simulink model "spoco6_250"  (R2013a)
settings: Solver=VariableStepDiscrete  SolverMode=SingleTasking  StartTime=0.0  StopTime=10.0  RelTol=1e-3
undefined symbols (not defined in the file or in its folder): casper_library_multipliers, cmult_4bit_em
libraries: xbsIndex_r4 x1937, xps_library x51, casper_library_misc x45, casper_library_sources x6
(part 8 of 23)

== system spoco6_250/xengine6/af ==
  a+bi : Inport
  c+di : Inport  Port=2
  new_acc : Inport  Port=3
  Counter : xbsIndex_r4/Counter  cnt_type=Free Running  cnt_to=Inf  operation=Up  start_count=0  cnt_by_val=1  arith_type=Unsigned  n_bits=nchan  bin_pt=0  load_pin=off  rst=on  en=on  explicit_period=on  period=1  use_behavioral_HDL=off  implementation=Fabric  dbl_ovrd=off  block_type=counter
  Delay : xbsIndex_r4/Delay  rst=off  infoeditControl=Selection of Reset will increase slice count due to use of real FFs and instead of SRLs  en=off  latency=mult_latency + add_latency  reg_retiming=off  dbl_ovrd=off  block_type=delay
  c_to_ri1 : casper_library_misc/c_to_ri  n_bits=n_bits  bin_pt=n_bits-1
      settings: AttributesFormatString=4_3 r/i
  c_to_ri2 : casper_library_misc/c_to_ri  n_bits=n_bits  bin_pt=n_bits-1
      settings: AttributesFormatString=4_3 r/i
  cmult_4bit_em* : Subsystem  AncestorBlock=casper_library_multipliers/cmult_4bit_em*  mask(cmult_4bit_em*){mult_latency=mult_latency, add_latency=add_latency}
      mask prompts: mult_latency "Mult Latency"; add_latency "Add Latency"
      mask help: Perform a conjugating complex multiplication (a+bi)(c-di)=(ac+bd)+(bc-ad)i. Implements the logic in dedicated multipliers.
      mask Help: eval('xlWeb(''http://casper.berkeley.edu/wiki/Cmult_4bit_em_'')')
  imag : xps_library/Shared BRAM  Tag=xps:bram  arith_type="Signed  (2's comp)"  addr_width=max(nchan,10)  data_width=32  reg_prim_output=off  reg_core_output=off  optimization=Minimum_Area  data_bin_pt=min(2*(n_bits-1), 30)  init_vals=0  sample_rate=1
  real : xps_library/Shared BRAM  Tag=xps:bram  arith_type="Signed  (2's comp)"  addr_width=max(nchan,10)  data_width=32  reg_prim_output=off  reg_core_output=off  optimization=Minimum_Area  data_bin_pt=min(2*(n_bits-1), 30)  init_vals=0  sample_rate=1
  simple_bram_vacc : Subsystem  AncestorBlock=casper_library_accumulators/simple_bram_vacc  mask(simple_bram_vacc){vec_len=2^nchan, arith_type=Signed, n_bits=32, bin_pt=30}
      mask prompts: vec_len "Vector length:"; arith_type "Output type:"; n_bits "Bit width (output):"; bin_pt "Binary point (output):"
      mask help: This simple vector accumulator is based on a shift register. It outputs its previous accumulated vector after a new_acc pulse is received.
      mask init:
      | simple_bram_vacc_init(gcb, ...
      |     'vec_len', vec_len, ...
      |     'arith_type', arith_type, ...
      |     'n_bits', n_bits, ...
      |     'bin_pt', bin_pt);
      mask TypeOptions arith_type: Signed | Unsigned
  simple_bram_vacc1 : Subsystem  AncestorBlock=casper_library_accumulators/simple_bram_vacc  mask(simple_bram_vacc){vec_len=2^nchan, arith_type=Signed, n_bits=32, bin_pt=30}
      mask prompts: vec_len "Vector length:"; arith_type "Output type:"; n_bits "Bit width (output):"; bin_pt "Binary point (output):"
      mask help: This simple vector accumulator is based on a shift register. It outputs its previous accumulated vector after a new_acc pulse is received.
      mask init:
      | simple_bram_vacc_init(gcb, ...
      |     'vec_len', vec_len, ...
      |     'arith_type', arith_type, ...
      |     'n_bits', n_bits, ...
      |     'bin_pt', bin_pt);
      mask TypeOptions arith_type: Signed | Unsigned
  wires:
  simple_bram_vacc1/2(valid) -> imag/3
  simple_bram_vacc1/1(dout) -> imag/2
  Delay/1 -> simple_bram_vacc1/1(new_acc), simple_bram_vacc/1(new_acc), Counter/1
  simple_bram_vacc/1(dout) -> real/2
  Counter/1 -> imag/1, real/1
  simple_bram_vacc/2(valid) -> Counter/2, real/3
  new_acc/1 -> Delay/1
  c+di/1 -> c_to_ri2/1
  a+bi/1 -> c_to_ri1/1
  c_to_ri1/1 -> cmult_4bit_em*/1(a)
  c_to_ri1/2 -> cmult_4bit_em*/2(b)
  c_to_ri2/2 -> cmult_4bit_em*/4(d)
  c_to_ri2/1 -> cmult_4bit_em*/3(c)
  cmult_4bit_em*/1(real) -> simple_bram_vacc/2(din)
  cmult_4bit_em*/2(imag) -> simple_bram_vacc1/2(din)

== system spoco6_250/xengine6/bb ==
  a+bi : Inport
  c+di : Inport  Port=2
  new_acc : Inport  Port=3
  Counter : xbsIndex_r4/Counter  cnt_type=Free Running  cnt_to=Inf  operation=Up  start_count=0  cnt_by_val=1  arith_type=Unsigned  n_bits=nchan  bin_pt=0  load_pin=off  rst=on  en=on  explicit_period=on  period=1  use_behavioral_HDL=off  implementation=Fabric  dbl_ovrd=off  block_type=counter
  Delay : xbsIndex_r4/Delay  rst=off  infoeditControl=Selection of Reset will increase slice count due to use of real FFs and instead of SRLs  en=off  latency=mult_latency + add_latency  reg_retiming=off  dbl_ovrd=off  block_type=delay
  c_to_ri1 : casper_library_misc/c_to_ri  n_bits=n_bits  bin_pt=n_bits-1
      settings: AttributesFormatString=4_3 r/i
  c_to_ri2 : casper_library_misc/c_to_ri  n_bits=n_bits  bin_pt=n_bits-1
      settings: AttributesFormatString=4_3 r/i
  cmult_4bit_em* : Subsystem  AncestorBlock=casper_library_multipliers/cmult_4bit_em*  mask(cmult_4bit_em*){mult_latency=mult_latency, add_latency=add_latency}
      mask prompts: mult_latency "Mult Latency"; add_latency "Add Latency"
      mask help: Perform a conjugating complex multiplication (a+bi)(c-di)=(ac+bd)+(bc-ad)i. Implements the logic in dedicated multipliers.
      mask Help: eval('xlWeb(''http://casper.berkeley.edu/wiki/Cmult_4bit_em_'')')
  real : xps_library/Shared BRAM  Tag=xps:bram  arith_type="Signed  (2's comp)"  addr_width=max(nchan,10)  data_width=32  reg_prim_output=off  reg_core_output=off  optimization=Minimum_Area  data_bin_pt=min(2*(n_bits-1), 30)  init_vals=0  sample_rate=1
  simple_bram_vacc : Subsystem  AncestorBlock=casper_library_accumulators/simple_bram_vacc  mask(simple_bram_vacc){vec_len=2^nchan, arith_type=Signed, n_bits=32, bin_pt=30}
      mask prompts: vec_len "Vector length:"; arith_type "Output type:"; n_bits "Bit width (output):"; bin_pt "Binary point (output):"
      mask help: This simple vector accumulator is based on a shift register. It outputs its previous accumulated vector after a new_acc pulse is received.
      mask init:
      | simple_bram_vacc_init(gcb, ...
      |     'vec_len', vec_len, ...
      |     'arith_type', arith_type, ...
      |     'n_bits', n_bits, ...
      |     'bin_pt', bin_pt);
      mask TypeOptions arith_type: Signed | Unsigned
  wires:
  c_to_ri2/1 -> cmult_4bit_em*/3(c)
  c_to_ri2/2 -> cmult_4bit_em*/4(d)
  c_to_ri1/2 -> cmult_4bit_em*/2(b)
  c_to_ri1/1 -> cmult_4bit_em*/1(a)
  Delay/1 -> simple_bram_vacc/1(new_acc), Counter/1
  simple_bram_vacc/1(dout) -> real/2
  Counter/1 -> real/1
  simple_bram_vacc/2(valid) -> real/3, Counter/2
  a+bi/1 -> c_to_ri1/1
  c+di/1 -> c_to_ri2/1
  new_acc/1 -> Delay/1
  cmult_4bit_em*/1(real) -> simple_bram_vacc/2(din)

== system spoco6_250/xengine6/bc ==
  a+bi : Inport
  c+di : Inport  Port=2
  new_acc : Inport  Port=3
  Counter : xbsIndex_r4/Counter  cnt_type=Free Running  cnt_to=Inf  operation=Up  start_count=0  cnt_by_val=1  arith_type=Unsigned  n_bits=nchan  bin_pt=0  load_pin=off  rst=on  en=on  explicit_period=on  period=1  use_behavioral_HDL=off  implementation=Fabric  dbl_ovrd=off  block_type=counter
  Delay : xbsIndex_r4/Delay  rst=off  infoeditControl=Selection of Reset will increase slice count due to use of real FFs and instead of SRLs  en=off  latency=mult_latency + add_latency  reg_retiming=off  dbl_ovrd=off  block_type=delay
  c_to_ri1 : casper_library_misc/c_to_ri  n_bits=n_bits  bin_pt=n_bits-1
      settings: AttributesFormatString=4_3 r/i
  c_to_ri2 : casper_library_misc/c_to_ri  n_bits=n_bits  bin_pt=n_bits-1
      settings: AttributesFormatString=4_3 r/i
  cmult_4bit_em* : Subsystem  AncestorBlock=casper_library_multipliers/cmult_4bit_em*  mask(cmult_4bit_em*){mult_latency=mult_latency, add_latency=add_latency}
      mask prompts: mult_latency "Mult Latency"; add_latency "Add Latency"
      mask help: Perform a conjugating complex multiplication (a+bi)(c-di)=(ac+bd)+(bc-ad)i. Implements the logic in dedicated multipliers.
      mask Help: eval('xlWeb(''http://casper.berkeley.edu/wiki/Cmult_4bit_em_'')')
  imag : xps_library/Shared BRAM  Tag=xps:bram  arith_type="Signed  (2's comp)"  addr_width=max(nchan,10)  data_width=32  reg_prim_output=off  reg_core_output=off  optimization=Minimum_Area  data_bin_pt=min(2*(n_bits-1), 30)  init_vals=0  sample_rate=1
  real : xps_library/Shared BRAM  Tag=xps:bram  arith_type="Signed  (2's comp)"  addr_width=max(nchan,10)  data_width=32  reg_prim_output=off  reg_core_output=off  optimization=Minimum_Area  data_bin_pt=min(2*(n_bits-1), 30)  init_vals=0  sample_rate=1
  simple_bram_vacc : Subsystem  AncestorBlock=casper_library_accumulators/simple_bram_vacc  mask(simple_bram_vacc){vec_len=2^nchan, arith_type=Signed, n_bits=32, bin_pt=30}
      mask prompts: vec_len "Vector length:"; arith_type "Output type:"; n_bits "Bit width (output):"; bin_pt "Binary point (output):"
      mask help: This simple vector accumulator is based on a shift register. It outputs its previous accumulated vector after a new_acc pulse is received.
      mask init:
      | simple_bram_vacc_init(gcb, ...
      |     'vec_len', vec_len, ...
      |     'arith_type', arith_type, ...
      |     'n_bits', n_bits, ...
      |     'bin_pt', bin_pt);
      mask TypeOptions arith_type: Signed | Unsigned
  simple_bram_vacc1 : Subsystem  AncestorBlock=casper_library_accumulators/simple_bram_vacc  mask(simple_bram_vacc){vec_len=2^nchan, arith_type=Signed, n_bits=32, bin_pt=30}
      mask prompts: vec_len "Vector length:"; arith_type "Output type:"; n_bits "Bit width (output):"; bin_pt "Binary point (output):"
      mask help: This simple vector accumulator is based on a shift register. It outputs its previous accumulated vector after a new_acc pulse is received.
      mask init:
      | simple_bram_vacc_init(gcb, ...
      |     'vec_len', vec_len, ...
      |     'arith_type', arith_type, ...
      |     'n_bits', n_bits, ...
      |     'bin_pt', bin_pt);
      mask TypeOptions arith_type: Signed | Unsigned
  wires:
  simple_bram_vacc1/2(valid) -> imag/3
  simple_bram_vacc1/1(dout) -> imag/2
  Delay/1 -> simple_bram_vacc1/1(new_acc), simple_bram_vacc/1(new_acc), Counter/1
  simple_bram_vacc/1(dout) -> real/2
  Counter/1 -> imag/1, real/1
  simple_bram_vacc/2(valid) -> Counter/2, real/3
  new_acc/1 -> Delay/1
  c+di/1 -> c_to_ri2/1
  a+bi/1 -> c_to_ri1/1
  c_to_ri1/1 -> cmult_4bit_em*/1(a)
  c_to_ri1/2 -> cmult_4bit_em*/2(b)
  c_to_ri2/2 -> cmult_4bit_em*/4(d)
  c_to_ri2/1 -> cmult_4bit_em*/3(c)
  cmult_4bit_em*/1(real) -> simple_bram_vacc/2(din)
  cmult_4bit_em*/2(imag) -> simple_bram_vacc1/2(din)

== system spoco6_250/xengine6/bd ==
  a+bi : Inport
  c+di : Inport  Port=2
  new_acc : Inport  Port=3
  Counter : xbsIndex_r4/Counter  cnt_type=Free Running  cnt_to=Inf  operation=Up  start_count=0  cnt_by_val=1  arith_type=Unsigned  n_bits=nchan  bin_pt=0  load_pin=off  rst=on  en=on  explicit_period=on  period=1  use_behavioral_HDL=off  implementation=Fabric  dbl_ovrd=off  block_type=counter
  Delay : xbsIndex_r4/Delay  rst=off  infoeditControl=Selection of Reset will increase slice count due to use of real FFs and instead of SRLs  en=off  latency=mult_latency + add_latency  reg_retiming=off  dbl_ovrd=off  block_type=delay
  c_to_ri1 : casper_library_misc/c_to_ri  n_bits=n_bits  bin_pt=n_bits-1
      settings: AttributesFormatString=4_3 r/i
  c_to_ri2 : casper_library_misc/c_to_ri  n_bits=n_bits  bin_pt=n_bits-1
      settings: AttributesFormatString=4_3 r/i
  cmult_4bit_em* : Subsystem  AncestorBlock=casper_library_multipliers/cmult_4bit_em*  mask(cmult_4bit_em*){mult_latency=mult_latency, add_latency=add_latency}
      mask prompts: mult_latency "Mult Latency"; add_latency "Add Latency"
      mask help: Perform a conjugating complex multiplication (a+bi)(c-di)=(ac+bd)+(bc-ad)i. Implements the logic in dedicated multipliers.
      mask Help: eval('xlWeb(''http://casper.berkeley.edu/wiki/Cmult_4bit_em_'')')
  imag : xps_library/Shared BRAM  Tag=xps:bram  arith_type="Signed  (2's comp)"  addr_width=max(nchan,10)  data_width=32  reg_prim_output=off  reg_core_output=off  optimization=Minimum_Area  data_bin_pt=min(2*(n_bits-1), 30)  init_vals=0  sample_rate=1
  real : xps_library/Shared BRAM  Tag=xps:bram  arith_type="Signed  (2's comp)"  addr_width=max(nchan,10)  data_width=32  reg_prim_output=off  reg_core_output=off  optimization=Minimum_Area  data_bin_pt=min(2*(n_bits-1), 30)  init_vals=0  sample_rate=1
  simple_bram_vacc : Subsystem  AncestorBlock=casper_library_accumulators/simple_bram_vacc  mask(simple_bram_vacc){vec_len=2^nchan, arith_type=Signed, n_bits=32, bin_pt=30}
      mask prompts: vec_len "Vector length:"; arith_type "Output type:"; n_bits "Bit width (output):"; bin_pt "Binary point (output):"
      mask help: This simple vector accumulator is based on a shift register. It outputs its previous accumulated vector after a new_acc pulse is received.
      mask init:
      | simple_bram_vacc_init(gcb, ...
      |     'vec_len', vec_len, ...
      |     'arith_type', arith_type, ...
      |     'n_bits', n_bits, ...
      |     'bin_pt', bin_pt);
      mask TypeOptions arith_type: Signed | Unsigned
  simple_bram_vacc1 : Subsystem  AncestorBlock=casper_library_accumulators/simple_bram_vacc  mask(simple_bram_vacc){vec_len=2^nchan, arith_type=Signed, n_bits=32, bin_pt=30}
      mask prompts: vec_len "Vector length:"; arith_type "Output type:"; n_bits "Bit width (output):"; bin_pt "Binary point (output):"
      mask help: This simple vector accumulator is based on a shift register. It outputs its previous accumulated vector after a new_acc pulse is received.
      mask init:
      | simple_bram_vacc_init(gcb, ...
      |     'vec_len', vec_len, ...
      |     'arith_type', arith_type, ...
      |     'n_bits', n_bits, ...
      |     'bin_pt', bin_pt);
      mask TypeOptions arith_type: Signed | Unsigned
  wires:
  cmult_4bit_em*/2(imag) -> simple_bram_vacc1/2(din)
  cmult_4bit_em*/1(real) -> simple_bram_vacc/2(din)
  c_to_ri2/1 -> cmult_4bit_em*/3(c)
  c_to_ri2/2 -> cmult_4bit_em*/4(d)
  c_to_ri1/2 -> cmult_4bit_em*/2(b)
  c_to_ri1/1 -> cmult_4bit_em*/1(a)
  a+bi/1 -> c_to_ri1/1
  c+di/1 -> c_to_ri2/1
  new_acc/1 -> Delay/1
  simple_bram_vacc/2(valid) -> real/3, Counter/2
  Counter/1 -> real/1, imag/1
  simple_bram_vacc/1(dout) -> real/2
  Delay/1 -> Counter/1, simple_bram_vacc/1(new_acc), simple_bram_vacc1/1(new_acc)
  simple_bram_vacc1/1(dout) -> imag/2
  simple_bram_vacc1/2(valid) -> imag/3

== system spoco6_250/xengine6/be ==
  a+bi : Inport
  c+di : Inport  Port=2
  new_acc : Inport  Port=3
  Counter : xbsIndex_r4/Counter  cnt_type=Free Running  cnt_to=Inf  operation=Up  start_count=0  cnt_by_val=1  arith_type=Unsigned  n_bits=nchan  bin_pt=0  load_pin=off  rst=on  en=on  explicit_period=on  period=1  use_behavioral_HDL=off  implementation=Fabric  dbl_ovrd=off  block_type=counter
  Delay : xbsIndex_r4/Delay  rst=off  infoeditControl=Selection of Reset will increase slice count due to use of real FFs and instead of SRLs  en=off  latency=mult_latency + add_latency  reg_retiming=off  dbl_ovrd=off  block_type=delay
  c_to_ri1 : casper_library_misc/c_to_ri  n_bits=n_bits  bin_pt=n_bits-1
      settings: AttributesFormatString=4_3 r/i
  c_to_ri2 : casper_library_misc/c_to_ri  n_bits=n_bits  bin_pt=n_bits-1
      settings: AttributesFormatString=4_3 r/i
  cmult_4bit_em* : Subsystem  AncestorBlock=casper_library_multipliers/cmult_4bit_em*  mask(cmult_4bit_em*){mult_latency=mult_latency, add_latency=add_latency}
      mask prompts: mult_latency "Mult Latency"; add_latency "Add Latency"
      mask help: Perform a conjugating complex multiplication (a+bi)(c-di)=(ac+bd)+(bc-ad)i. Implements the logic in dedicated multipliers.
      mask Help: eval('xlWeb(''http://casper.berkeley.edu/wiki/Cmult_4bit_em_'')')
  imag : xps_library/Shared BRAM  Tag=xps:bram  arith_type="Signed  (2's comp)"  addr_width=max(nchan,10)  data_width=32  reg_prim_output=off  reg_core_output=off  optimization=Minimum_Area  data_bin_pt=min(2*(n_bits-1), 30)  init_vals=0  sample_rate=1
  real : xps_library/Shared BRAM  Tag=xps:bram  arith_type="Signed  (2's comp)"  addr_width=max(nchan,10)  data_width=32  reg_prim_output=off  reg_core_output=off  optimization=Minimum_Area  data_bin_pt=min(2*(n_bits-1), 30)  init_vals=0  sample_rate=1
  simple_bram_vacc : Subsystem  AncestorBlock=casper_library_accumulators/simple_bram_vacc  mask(simple_bram_vacc){vec_len=2^nchan, arith_type=Signed, n_bits=32, bin_pt=30}
      mask prompts: vec_len "Vector length:"; arith_type "Output type:"; n_bits "Bit width (output):"; bin_pt "Binary point (output):"
      mask help: This simple vector accumulator is based on a shift register. It outputs its previous accumulated vector after a new_acc pulse is received.
      mask init:
      | simple_bram_vacc_init(gcb, ...
      |     'vec_len', vec_len, ...
      |     'arith_type', arith_type, ...
      |     'n_bits', n_bits, ...
      |     'bin_pt', bin_pt);
      mask TypeOptions arith_type: Signed | Unsigned
  simple_bram_vacc1 : Subsystem  AncestorBlock=casper_library_accumulators/simple_bram_vacc  mask(simple_bram_vacc){vec_len=2^nchan, arith_type=Signed, n_bits=32, bin_pt=30}
      mask prompts: vec_len "Vector length:"; arith_type "Output type:"; n_bits "Bit width (output):"; bin_pt "Binary point (output):"
      mask help: This simple vector accumulator is based on a shift register. It outputs its previous accumulated vector after a new_acc pulse is received.
      mask init:
      | simple_bram_vacc_init(gcb, ...
      |     'vec_len', vec_len, ...
      |     'arith_type', arith_type, ...
      |     'n_bits', n_bits, ...
      |     'bin_pt', bin_pt);
      mask TypeOptions arith_type: Signed | Unsigned
  wires:
  simple_bram_vacc1/2(valid) -> imag/3
  simple_bram_vacc1/1(dout) -> imag/2
  Delay/1 -> simple_bram_vacc1/1(new_acc), simple_bram_vacc/1(new_acc), Counter/1
  simple_bram_vacc/1(dout) -> real/2
  Counter/1 -> imag/1, real/1
  simple_bram_vacc/2(valid) -> Counter/2, real/3
  new_acc/1 -> Delay/1
  c+di/1 -> c_to_ri2/1
  a+bi/1 -> c_to_ri1/1
  c_to_ri1/1 -> cmult_4bit_em*/1(a)
  c_to_ri1/2 -> cmult_4bit_em*/2(b)
  c_to_ri2/2 -> cmult_4bit_em*/4(d)
  c_to_ri2/1 -> cmult_4bit_em*/3(c)
  cmult_4bit_em*/1(real) -> simple_bram_vacc/2(din)
  cmult_4bit_em*/2(imag) -> simple_bram_vacc1/2(din)

== system spoco6_250/xengine6/bf ==
  a+bi : Inport
  c+di : Inport  Port=2
  new_acc : Inport  Port=3
  Counter : xbsIndex_r4/Counter  cnt_type=Free Running  cnt_to=Inf  operation=Up  start_count=0  cnt_by_val=1  arith_type=Unsigned  n_bits=nchan  bin_pt=0  load_pin=off  rst=on  en=on  explicit_period=on  period=1  use_behavioral_HDL=off  implementation=Fabric  dbl_ovrd=off  block_type=counter
  Delay : xbsIndex_r4/Delay  rst=off  infoeditControl=Selection of Reset will increase slice count due to use of real FFs and instead of SRLs  en=off  latency=mult_latency + add_latency  reg_retiming=off  dbl_ovrd=off  block_type=delay
  c_to_ri1 : casper_library_misc/c_to_ri  n_bits=n_bits  bin_pt=n_bits-1
      settings: AttributesFormatString=4_3 r/i
  c_to_ri2 : casper_library_misc/c_to_ri  n_bits=n_bits  bin_pt=n_bits-1
      settings: AttributesFormatString=4_3 r/i
  cmult_4bit_em* : Subsystem  AncestorBlock=casper_library_multipliers/cmult_4bit_em*  mask(cmult_4bit_em*){mult_latency=mult_latency, add_latency=add_latency}
      mask prompts: mult_latency "Mult Latency"; add_latency "Add Latency"
      mask help: Perform a conjugating complex multiplication (a+bi)(c-di)=(ac+bd)+(bc-ad)i. Implements the logic in dedicated multipliers.
      mask Help: eval('xlWeb(''http://casper.berkeley.edu/wiki/Cmult_4bit_em_'')')
  imag : xps_library/Shared BRAM  Tag=xps:bram  arith_type="Signed  (2's comp)"  addr_width=max(nchan,10)  data_width=32  reg_prim_output=off  reg_core_output=off  optimization=Minimum_Area  data_bin_pt=min(2*(n_bits-1), 30)  init_vals=0  sample_rate=1
  real : xps_library/Shared BRAM  Tag=xps:bram  arith_type="Signed  (2's comp)"  addr_width=max(nchan,10)  data_width=32  reg_prim_output=off  reg_core_output=off  optimization=Minimum_Area  data_bin_pt=min(2*(n_bits-1), 30)  init_vals=0  sample_rate=1
  simple_bram_vacc : Subsystem  AncestorBlock=casper_library_accumulators/simple_bram_vacc  mask(simple_bram_vacc){vec_len=2^nchan, arith_type=Signed, n_bits=32, bin_pt=30}
      mask prompts: vec_len "Vector length:"; arith_type "Output type:"; n_bits "Bit width (output):"; bin_pt "Binary point (output):"
      mask help: This simple vector accumulator is based on a shift register. It outputs its previous accumulated vector after a new_acc pulse is received.
      mask init:
      | simple_bram_vacc_init(gcb, ...
      |     'vec_len', vec_len, ...
      |     'arith_type', arith_type, ...
      |     'n_bits', n_bits, ...
      |     'bin_pt', bin_pt);
      mask TypeOptions arith_type: Signed | Unsigned
  simple_bram_vacc1 : Subsystem  AncestorBlock=casper_library_accumulators/simple_bram_vacc  mask(simple_bram_vacc){vec_len=2^nchan, arith_type=Signed, n_bits=32, bin_pt=30}
      mask prompts: vec_len "Vector length:"; arith_type "Output type:"; n_bits "Bit width (output):"; bin_pt "Binary point (output):"
      mask help: This simple vector accumulator is based on a shift register. It outputs its previous accumulated vector after a new_acc pulse is received.
      mask init:
      | simple_bram_vacc_init(gcb, ...
      |     'vec_len', vec_len, ...
      |     'arith_type', arith_type, ...
      |     'n_bits', n_bits, ...
      |     'bin_pt', bin_pt);
      mask TypeOptions arith_type: Signed | Unsigned
  wires:
  cmult_4bit_em*/2(imag) -> simple_bram_vacc1/2(din)
  cmult_4bit_em*/1(real) -> simple_bram_vacc/2(din)
  c_to_ri2/1 -> cmult_4bit_em*/3(c)
  c_to_ri2/2 -> cmult_4bit_em*/4(d)
  c_to_ri1/2 -> cmult_4bit_em*/2(b)
  c_to_ri1/1 -> cmult_4bit_em*/1(a)
  a+bi/1 -> c_to_ri1/1
  c+di/1 -> c_to_ri2/1
  new_acc/1 -> Delay/1
  simple_bram_vacc/2(valid) -> real/3, Counter/2
  Counter/1 -> real/1, imag/1
  simple_bram_vacc/1(dout) -> real/2
  Delay/1 -> Counter/1, simple_bram_vacc/1(new_acc), simple_bram_vacc1/1(new_acc)
  simple_bram_vacc1/1(dout) -> imag/2
  simple_bram_vacc1/2(valid) -> imag/3

== system spoco6_250/xengine6/bus_expand ==
  bus_in : Inport
  reinterpret{1..6} (6 alike) : xbsIndex_r4/Reinterpret  force_arith_type=on  arith_type=Unsigned  force_bin_pt=on  bin_pt=0  block_type=reinterpret
  slice1 : xbsIndex_r4/Slice  nbits=8  boolean_output=off  mode=Upper Bit Location + Width  bit1=-40  base1=MSB of Input  bit0=0  base0=LSB of Input  dbl_ovrd=off  block_type=slice
  slice2 : xbsIndex_r4/Slice  nbits=8  boolean_output=off  mode=Upper Bit Location + Width  bit1=-32  base1=MSB of Input  bit0=0  base0=LSB of Input  dbl_ovrd=off  block_type=slice
  slice3 : xbsIndex_r4/Slice  nbits=8  boolean_output=off  mode=Upper Bit Location + Width  bit1=-24  base1=MSB of Input  bit0=0  base0=LSB of Input  dbl_ovrd=off  block_type=slice
  slice4 : xbsIndex_r4/Slice  nbits=8  boolean_output=off  mode=Upper Bit Location + Width  bit1=-16  base1=MSB of Input  bit0=0  base0=LSB of Input  dbl_ovrd=off  block_type=slice
  slice5 : xbsIndex_r4/Slice  nbits=8  boolean_output=off  mode=Upper Bit Location + Width  bit1=-8  base1=MSB of Input  bit0=0  base0=LSB of Input  dbl_ovrd=off  block_type=slice
  slice6 : xbsIndex_r4/Slice  nbits=8  boolean_output=off  mode=Upper Bit Location + Width  bit1=0  base1=MSB of Input  bit0=0  base0=LSB of Input  dbl_ovrd=off  block_type=slice
  msb_out6 : Outport
  out5 : Outport  Port=2
  out4 : Outport  Port=3
  out3 : Outport  Port=4
  out2 : Outport  Port=5
  lsb_out1 : Outport  Port=6
  wires:
  bus_in/1 -> slice6/1, slice5/1, slice4/1, slice3/1, slice2/1, slice1/1
  slice6/1 -> reinterpret6/1
  reinterpret6/1 -> msb_out6/1
  slice5/1 -> reinterpret5/1
  reinterpret5/1 -> out5/1
  slice4/1 -> reinterpret4/1
  reinterpret4/1 -> out4/1
  slice3/1 -> reinterpret3/1
  reinterpret3/1 -> out3/1
  slice2/1 -> reinterpret2/1
  reinterpret2/1 -> out2/1
  slice1/1 -> reinterpret1/1
  reinterpret1/1 -> lsb_out1/1

== system spoco6_250/xengine6/cc ==
  a+bi : Inport
  c+di : Inport  Port=2
  new_acc : Inport  Port=3
  Counter : xbsIndex_r4/Counter  cnt_type=Free Running  cnt_to=Inf  operation=Up  start_count=0  cnt_by_val=1  arith_type=Unsigned  n_bits=nchan  bin_pt=0  load_pin=off  rst=on  en=on  explicit_period=on  period=1  use_behavioral_HDL=off  implementation=Fabric  dbl_ovrd=off  block_type=counter
  Delay : xbsIndex_r4/Delay  rst=off  infoeditControl=Selection of Reset will increase slice count due to use of real FFs and instead of SRLs  en=off  latency=mult_latency + add_latency  reg_retiming=off  dbl_ovrd=off  block_type=delay
  c_to_ri1 : casper_library_misc/c_to_ri  n_bits=n_bits  bin_pt=n_bits-1
      settings: AttributesFormatString=4_3 r/i
  c_to_ri2 : casper_library_misc/c_to_ri  n_bits=n_bits  bin_pt=n_bits-1
      settings: AttributesFormatString=4_3 r/i
  cmult_4bit_em* : Subsystem  AncestorBlock=casper_library_multipliers/cmult_4bit_em*  mask(cmult_4bit_em*){mult_latency=mult_latency, add_latency=add_latency}
      mask prompts: mult_latency "Mult Latency"; add_latency "Add Latency"
      mask help: Perform a conjugating complex multiplication (a+bi)(c-di)=(ac+bd)+(bc-ad)i. Implements the logic in dedicated multipliers.
      mask Help: eval('xlWeb(''http://casper.berkeley.edu/wiki/Cmult_4bit_em_'')')
  real : xps_library/Shared BRAM  Tag=xps:bram  arith_type="Signed  (2's comp)"  addr_width=max(nchan,10)  data_width=32  reg_prim_output=off  reg_core_output=off  optimization=Minimum_Area  data_bin_pt=min(2*(n_bits-1), 30)  init_vals=0  sample_rate=1
  simple_bram_vacc : Subsystem  AncestorBlock=casper_library_accumulators/simple_bram_vacc  mask(simple_bram_vacc){vec_len=2^nchan, arith_type=Signed, n_bits=32, bin_pt=30}
      mask prompts: vec_len "Vector length:"; arith_type "Output type:"; n_bits "Bit width (output):"; bin_pt "Binary point (output):"
      mask help: This simple vector accumulator is based on a shift register. It outputs its previous accumulated vector after a new_acc pulse is received.
      mask init:
      | simple_bram_vacc_init(gcb, ...
      |     'vec_len', vec_len, ...
      |     'arith_type', arith_type, ...
      |     'n_bits', n_bits, ...
      |     'bin_pt', bin_pt);
      mask TypeOptions arith_type: Signed | Unsigned
  wires:
  cmult_4bit_em*/1(real) -> simple_bram_vacc/2(din)
  new_acc/1 -> Delay/1
  c+di/1 -> c_to_ri2/1
  a+bi/1 -> c_to_ri1/1
  simple_bram_vacc/2(valid) -> Counter/2, real/3
  Counter/1 -> real/1
  simple_bram_vacc/1(dout) -> real/2
  Delay/1 -> Counter/1, simple_bram_vacc/1(new_acc)
  c_to_ri1/1 -> cmult_4bit_em*/1(a)
  c_to_ri1/2 -> cmult_4bit_em*/2(b)
  c_to_ri2/2 -> cmult_4bit_em*/4(d)
  c_to_ri2/1 -> cmult_4bit_em*/3(c)

== system spoco6_250/xengine6/cd ==
  a+bi : Inport
  c+di : Inport  Port=2
  new_acc : Inport  Port=3
  Counter : xbsIndex_r4/Counter  cnt_type=Free Running  cnt_to=Inf  operation=Up  start_count=0  cnt_by_val=1  arith_type=Unsigned  n_bits=nchan  bin_pt=0  load_pin=off  rst=on  en=on  explicit_period=on  period=1  use_behavioral_HDL=off  implementation=Fabric  dbl_ovrd=off  block_type=counter
  Delay : xbsIndex_r4/Delay  rst=off  infoeditControl=Selection of Reset will increase slice count due to use of real FFs and instead of SRLs  en=off  latency=mult_latency + add_latency  reg_retiming=off  dbl_ovrd=off  block_type=delay
  c_to_ri1 : casper_library_misc/c_to_ri  n_bits=n_bits  bin_pt=n_bits-1
      settings: AttributesFormatString=4_3 r/i
  c_to_ri2 : casper_library_misc/c_to_ri  n_bits=n_bits  bin_pt=n_bits-1
      settings: AttributesFormatString=4_3 r/i
  cmult_4bit_em* : Subsystem  AncestorBlock=casper_library_multipliers/cmult_4bit_em*  mask(cmult_4bit_em*){mult_latency=mult_latency, add_latency=add_latency}
      mask prompts: mult_latency "Mult Latency"; add_latency "Add Latency"
      mask help: Perform a conjugating complex multiplication (a+bi)(c-di)=(ac+bd)+(bc-ad)i. Implements the logic in dedicated multipliers.
      mask Help: eval('xlWeb(''http://casper.berkeley.edu/wiki/Cmult_4bit_em_'')')
  imag : xps_library/Shared BRAM  Tag=xps:bram  arith_type="Signed  (2's comp)"  addr_width=max(nchan,10)  data_width=32  reg_prim_output=off  reg_core_output=off  optimization=Minimum_Area  data_bin_pt=min(2*(n_bits-1), 30)  init_vals=0  sample_rate=1
  real : xps_library/Shared BRAM  Tag=xps:bram  arith_type="Signed  (2's comp)"  addr_width=max(nchan,10)  data_width=32  reg_prim_output=off  reg_core_output=off  optimization=Minimum_Area  data_bin_pt=min(2*(n_bits-1), 30)  init_vals=0  sample_rate=1
  simple_bram_vacc : Subsystem  AncestorBlock=casper_library_accumulators/simple_bram_vacc  mask(simple_bram_vacc){vec_len=2^nchan, arith_type=Signed, n_bits=32, bin_pt=30}
      mask prompts: vec_len "Vector length:"; arith_type "Output type:"; n_bits "Bit width (output):"; bin_pt "Binary point (output):"
      mask help: This simple vector accumulator is based on a shift register. It outputs its previous accumulated vector after a new_acc pulse is received.
      mask init:
      | simple_bram_vacc_init(gcb, ...
      |     'vec_len', vec_len, ...
      |     'arith_type', arith_type, ...
      |     'n_bits', n_bits, ...
      |     'bin_pt', bin_pt);
      mask TypeOptions arith_type: Signed | Unsigned
  simple_bram_vacc1 : Subsystem  AncestorBlock=casper_library_accumulators/simple_bram_vacc  mask(simple_bram_vacc){vec_len=2^nchan, arith_type=Signed, n_bits=32, bin_pt=30}
      mask prompts: vec_len "Vector length:"; arith_type "Output type:"; n_bits "Bit width (output):"; bin_pt "Binary point (output):"
      mask help: This simple vector accumulator is based on a shift register. It outputs its previous accumulated vector after a new_acc pulse is received.
      mask init:
      | simple_bram_vacc_init(gcb, ...
      |     'vec_len', vec_len, ...
      |     'arith_type', arith_type, ...
      |     'n_bits', n_bits, ...
      |     'bin_pt', bin_pt);
      mask TypeOptions arith_type: Signed | Unsigned
  wires:
  simple_bram_vacc1/2(valid) -> imag/3
  simple_bram_vacc1/1(dout) -> imag/2
  Delay/1 -> simple_bram_vacc1/1(new_acc), simple_bram_vacc/1(new_acc), Counter/1
  simple_bram_vacc/1(dout) -> real/2
  Counter/1 -> imag/1, real/1
  simple_bram_vacc/2(valid) -> Counter/2, real/3
  new_acc/1 -> Delay/1
  c+di/1 -> c_to_ri2/1
  a+bi/1 -> c_to_ri1/1
  c_to_ri1/1 -> cmult_4bit_em*/1(a)
  c_to_ri1/2 -> cmult_4bit_em*/2(b)
  c_to_ri2/2 -> cmult_4bit_em*/4(d)
  c_to_ri2/1 -> cmult_4bit_em*/3(c)
  cmult_4bit_em*/1(real) -> simple_bram_vacc/2(din)
  cmult_4bit_em*/2(imag) -> simple_bram_vacc1/2(din)

== system spoco6_250/xengine6/ce ==
  a+bi : Inport
  c+di : Inport  Port=2
  new_acc : Inport  Port=3
  Counter : xbsIndex_r4/Counter  cnt_type=Free Running  cnt_to=Inf  operation=Up  start_count=0  cnt_by_val=1  arith_type=Unsigned  n_bits=nchan  bin_pt=0  load_pin=off  rst=on  en=on  explicit_period=on  period=1  use_behavioral_HDL=off  implementation=Fabric  dbl_ovrd=off  block_type=counter
  Delay : xbsIndex_r4/Delay  rst=off  infoeditControl=Selection of Reset will increase slice count due to use of real FFs and instead of SRLs  en=off  latency=mult_latency + add_latency  reg_retiming=off  dbl_ovrd=off  block_type=delay
  c_to_ri1 : casper_library_misc/c_to_ri  n_bits=n_bits  bin_pt=n_bits-1
      settings: AttributesFormatString=4_3 r/i
  c_to_ri2 : casper_library_misc/c_to_ri  n_bits=n_bits  bin_pt=n_bits-1
      settings: AttributesFormatString=4_3 r/i
  cmult_4bit_em* : Subsystem  AncestorBlock=casper_library_multipliers/cmult_4bit_em*  mask(cmult_4bit_em*){mult_latency=mult_latency, add_latency=add_latency}
      mask prompts: mult_latency "Mult Latency"; add_latency "Add Latency"
      mask help: Perform a conjugating complex multiplication (a+bi)(c-di)=(ac+bd)+(bc-ad)i. Implements the logic in dedicated multipliers.
      mask Help: eval('xlWeb(''http://casper.berkeley.edu/wiki/Cmult_4bit_em_'')')
  imag : xps_library/Shared BRAM  Tag=xps:bram  arith_type="Signed  (2's comp)"  addr_width=max(nchan,10)  data_width=32  reg_prim_output=off  reg_core_output=off  optimization=Minimum_Area  data_bin_pt=min(2*(n_bits-1), 30)  init_vals=0  sample_rate=1
  real : xps_library/Shared BRAM  Tag=xps:bram  arith_type="Signed  (2's comp)"  addr_width=max(nchan,10)  data_width=32  reg_prim_output=off  reg_core_output=off  optimization=Minimum_Area  data_bin_pt=min(2*(n_bits-1), 30)  init_vals=0  sample_rate=1
  simple_bram_vacc : Subsystem  AncestorBlock=casper_library_accumulators/simple_bram_vacc  mask(simple_bram_vacc){vec_len=2^nchan, arith_type=Signed, n_bits=32, bin_pt=30}
      mask prompts: vec_len "Vector length:"; arith_type "Output type:"; n_bits "Bit width (output):"; bin_pt "Binary point (output):"
      mask help: This simple vector accumulator is based on a shift register. It outputs its previous accumulated vector after a new_acc pulse is received.
      mask init:
      | simple_bram_vacc_init(gcb, ...
      |     'vec_len', vec_len, ...
      |     'arith_type', arith_type, ...
      |     'n_bits', n_bits, ...
      |     'bin_pt', bin_pt);
      mask TypeOptions arith_type: Signed | Unsigned
  simple_bram_vacc1 : Subsystem  AncestorBlock=casper_library_accumulators/simple_bram_vacc  mask(simple_bram_vacc){vec_len=2^nchan, arith_type=Signed, n_bits=32, bin_pt=30}
      mask prompts: vec_len "Vector length:"; arith_type "Output type:"; n_bits "Bit width (output):"; bin_pt "Binary point (output):"
      mask help: This simple vector accumulator is based on a shift register. It outputs its previous accumulated vector after a new_acc pulse is received.
      mask init:
      | simple_bram_vacc_init(gcb, ...
      |     'vec_len', vec_len, ...
      |     'arith_type', arith_type, ...
      |     'n_bits', n_bits, ...
      |     'bin_pt', bin_pt);
      mask TypeOptions arith_type: Signed | Unsigned
  wires:
  cmult_4bit_em*/2(imag) -> simple_bram_vacc1/2(din)
  cmult_4bit_em*/1(real) -> simple_bram_vacc/2(din)
  c_to_ri2/1 -> cmult_4bit_em*/3(c)
  c_to_ri2/2 -> cmult_4bit_em*/4(d)
  c_to_ri1/2 -> cmult_4bit_em*/2(b)
  c_to_ri1/1 -> cmult_4bit_em*/1(a)
  a+bi/1 -> c_to_ri1/1
  c+di/1 -> c_to_ri2/1
  new_acc/1 -> Delay/1
  simple_bram_vacc/2(valid) -> real/3, Counter/2
  Counter/1 -> real/1, imag/1
  simple_bram_vacc/1(dout) -> real/2
  Delay/1 -> Counter/1, simple_bram_vacc/1(new_acc), simple_bram_vacc1/1(new_acc)
  simple_bram_vacc1/1(dout) -> imag/2
  simple_bram_vacc1/2(valid) -> imag/3

== system spoco6_250/xengine6/cf ==
  a+bi : Inport
  c+di : Inport  Port=2
  new_acc : Inport  Port=3
  Counter : xbsIndex_r4/Counter  cnt_type=Free Running  cnt_to=Inf  operation=Up  start_count=0  cnt_by_val=1  arith_type=Unsigned  n_bits=nchan  bin_pt=0  load_pin=off  rst=on  en=on  explicit_period=on  period=1  use_behavioral_HDL=off  implementation=Fabric  dbl_ovrd=off  block_type=counter
  Delay : xbsIndex_r4/Delay  rst=off  infoeditControl=Selection of Reset will increase slice count due to use of real FFs and instead of SRLs  en=off  latency=mult_latency + add_latency  reg_retiming=off  dbl_ovrd=off  block_type=delay
  c_to_ri1 : casper_library_misc/c_to_ri  n_bits=n_bits  bin_pt=n_bits-1
      settings: AttributesFormatString=4_3 r/i
  c_to_ri2 : casper_library_misc/c_to_ri  n_bits=n_bits  bin_pt=n_bits-1
      settings: AttributesFormatString=4_3 r/i
  cmult_4bit_em* : Subsystem  AncestorBlock=casper_library_multipliers/cmult_4bit_em*  mask(cmult_4bit_em*){mult_latency=mult_latency, add_latency=add_latency}
      mask prompts: mult_latency "Mult Latency"; add_latency "Add Latency"
      mask help: Perform a conjugating complex multiplication (a+bi)(c-di)=(ac+bd)+(bc-ad)i. Implements the logic in dedicated multipliers.
      mask Help: eval('xlWeb(''http://casper.berkeley.edu/wiki/Cmult_4bit_em_'')')
  imag : xps_library/Shared BRAM  Tag=xps:bram  arith_type="Signed  (2's comp)"  addr_width=max(nchan,10)  data_width=32  reg_prim_output=off  reg_core_output=off  optimization=Minimum_Area  data_bin_pt=min(2*(n_bits-1), 30)  init_vals=0  sample_rate=1
  real : xps_library/Shared BRAM  Tag=xps:bram  arith_type="Signed  (2's comp)"  addr_width=max(nchan,10)  data_width=32  reg_prim_output=off  reg_core_output=off  optimization=Minimum_Area  data_bin_pt=min(2*(n_bits-1), 30)  init_vals=0  sample_rate=1
  simple_bram_vacc : Subsystem  AncestorBlock=casper_library_accumulators/simple_bram_vacc  mask(simple_bram_vacc){vec_len=2^nchan, arith_type=Signed, n_bits=32, bin_pt=30}
      mask prompts: vec_len "Vector length:"; arith_type "Output type:"; n_bits "Bit width (output):"; bin_pt "Binary point (output):"
      mask help: This simple vector accumulator is based on a shift register. It outputs its previous accumulated vector after a new_acc pulse is received.
      mask init:
      | simple_bram_vacc_init(gcb, ...
      |     'vec_len', vec_len, ...
      |     'arith_type', arith_type, ...
      |     'n_bits', n_bits, ...
      |     'bin_pt', bin_pt);
      mask TypeOptions arith_type: Signed | Unsigned
  simple_bram_vacc1 : Subsystem  AncestorBlock=casper_library_accumulators/simple_bram_vacc  mask(simple_bram_vacc){vec_len=2^nchan, arith_type=Signed, n_bits=32, bin_pt=30}
      mask prompts: vec_len "Vector length:"; arith_type "Output type:"; n_bits "Bit width (output):"; bin_pt "Binary point (output):"
      mask help: This simple vector accumulator is based on a shift register. It outputs its previous accumulated vector after a new_acc pulse is received.
      mask init:
      | simple_bram_vacc_init(gcb, ...
      |     'vec_len', vec_len, ...
      |     'arith_type', arith_type, ...
      |     'n_bits', n_bits, ...
      |     'bin_pt', bin_pt);
      mask TypeOptions arith_type: Signed | Unsigned
  wires:
  simple_bram_vacc1/2(valid) -> imag/3
  simple_bram_vacc1/1(dout) -> imag/2
  Delay/1 -> simple_bram_vacc1/1(new_acc), simple_bram_vacc/1(new_acc), Counter/1
  simple_bram_vacc/1(dout) -> real/2
  Counter/1 -> imag/1, real/1
  simple_bram_vacc/2(valid) -> Counter/2, real/3
  new_acc/1 -> Delay/1
  c+di/1 -> c_to_ri2/1
  a+bi/1 -> c_to_ri1/1
  c_to_ri1/1 -> cmult_4bit_em*/1(a)
  c_to_ri1/2 -> cmult_4bit_em*/2(b)
  c_to_ri2/2 -> cmult_4bit_em*/4(d)
  c_to_ri2/1 -> cmult_4bit_em*/3(c)
  cmult_4bit_em*/1(real) -> simple_bram_vacc/2(din)
  cmult_4bit_em*/2(imag) -> simple_bram_vacc1/2(din)

== system spoco6_250/xengine6/dd ==
  a+bi : Inport
  c+di : Inport  Port=2
  new_acc : Inport  Port=3
  Counter : xbsIndex_r4/Counter  cnt_type=Free Running  cnt_to=Inf  operation=Up  start_count=0  cnt_by_val=1  arith_type=Unsigned  n_bits=nchan  bin_pt=0  load_pin=off  rst=on  en=on  explicit_period=on  period=1  use_behavioral_HDL=off  implementation=Fabric  dbl_ovrd=off  block_type=counter
  Delay : xbsIndex_r4/Delay  rst=off  infoeditControl=Selection of Reset will increase slice count due to use of real FFs and instead of SRLs  en=off  latency=mult_latency + add_latency  reg_retiming=off  dbl_ovrd=off  block_type=delay
  c_to_ri1 : casper_library_misc/c_to_ri  n_bits=n_bits  bin_pt=n_bits-1
      settings: AttributesFormatString=4_3 r/i
  c_to_ri2 : casper_library_misc/c_to_ri  n_bits=n_bits  bin_pt=n_bits-1
      settings: AttributesFormatString=4_3 r/i
  cmult_4bit_em* : Subsystem  AncestorBlock=casper_library_multipliers/cmult_4bit_em*  mask(cmult_4bit_em*){mult_latency=mult_latency, add_latency=add_latency}
      mask prompts: mult_latency "Mult Latency"; add_latency "Add Latency"
      mask help: Perform a conjugating complex multiplication (a+bi)(c-di)=(ac+bd)+(bc-ad)i. Implements the logic in dedicated multipliers.
      mask Help: eval('xlWeb(''http://casper.berkeley.edu/wiki/Cmult_4bit_em_'')')
  real : xps_library/Shared BRAM  Tag=xps:bram  arith_type="Signed  (2's comp)"  addr_width=max(nchan,10)  data_width=32  reg_prim_output=off  reg_core_output=off  optimization=Minimum_Area  data_bin_pt=min(2*(n_bits-1), 30)  init_vals=0  sample_rate=1
  simple_bram_vacc : Subsystem  AncestorBlock=casper_library_accumulators/simple_bram_vacc  mask(simple_bram_vacc){vec_len=2^nchan, arith_type=Signed, n_bits=32, bin_pt=30}
      mask prompts: vec_len "Vector length:"; arith_type "Output type:"; n_bits "Bit width (output):"; bin_pt "Binary point (output):"
      mask help: This simple vector accumulator is based on a shift register. It outputs its previous accumulated vector after a new_acc pulse is received.
      mask init:
      | simple_bram_vacc_init(gcb, ...
      |     'vec_len', vec_len, ...
      |     'arith_type', arith_type, ...
      |     'n_bits', n_bits, ...
      |     'bin_pt', bin_pt);
      mask TypeOptions arith_type: Signed | Unsigned
  wires:
  c_to_ri2/1 -> cmult_4bit_em*/3(c)
  c_to_ri2/2 -> cmult_4bit_em*/4(d)
  c_to_ri1/2 -> cmult_4bit_em*/2(b)
  c_to_ri1/1 -> cmult_4bit_em*/1(a)
  Delay/1 -> simple_bram_vacc/1(new_acc), Counter/1
  simple_bram_vacc/1(dout) -> real/2
  Counter/1 -> real/1
  simple_bram_vacc/2(valid) -> real/3, Counter/2
  a+bi/1 -> c_to_ri1/1
  c+di/1 -> c_to_ri2/1
  new_acc/1 -> Delay/1
  cmult_4bit_em*/1(real) -> simple_bram_vacc/2(din)

== system spoco6_250/xengine6/de ==
  a+bi : Inport
  c+di : Inport  Port=2
  new_acc : Inport  Port=3
  Counter : xbsIndex_r4/Counter  cnt_type=Free Running  cnt_to=Inf  operation=Up  start_count=0  cnt_by_val=1  arith_type=Unsigned  n_bits=nchan  bin_pt=0  load_pin=off  rst=on  en=on  explicit_period=on  period=1  use_behavioral_HDL=off  implementation=Fabric  dbl_ovrd=off  block_type=counter
  Delay : xbsIndex_r4/Delay  rst=off  infoeditControl=Selection of Reset will increase slice count due to use of real FFs and instead of SRLs  en=off  latency=mult_latency + add_latency  reg_retiming=off  dbl_ovrd=off  block_type=delay
  c_to_ri1 : casper_library_misc/c_to_ri  n_bits=n_bits  bin_pt=n_bits-1
      settings: AttributesFormatString=4_3 r/i
  c_to_ri2 : casper_library_misc/c_to_ri  n_bits=n_bits  bin_pt=n_bits-1
      settings: AttributesFormatString=4_3 r/i
  cmult_4bit_em* : Subsystem  AncestorBlock=casper_library_multipliers/cmult_4bit_em*  mask(cmult_4bit_em*){mult_latency=mult_latency, add_latency=add_latency}
      mask prompts: mult_latency "Mult Latency"; add_latency "Add Latency"
      mask help: Perform a conjugating complex multiplication (a+bi)(c-di)=(ac+bd)+(bc-ad)i. Implements the logic in dedicated multipliers.
      mask Help: eval('xlWeb(''http://casper.berkeley.edu/wiki/Cmult_4bit_em_'')')
  imag : xps_library/Shared BRAM  Tag=xps:bram  arith_type="Signed  (2's comp)"  addr_width=max(nchan,10)  data_width=32  reg_prim_output=off  reg_core_output=off  optimization=Minimum_Area  data_bin_pt=min(2*(n_bits-1), 30)  init_vals=0  sample_rate=1
  real : xps_library/Shared BRAM  Tag=xps:bram  arith_type="Signed  (2's comp)"  addr_width=max(nchan,10)  data_width=32  reg_prim_output=off  reg_core_output=off  optimization=Minimum_Area  data_bin_pt=min(2*(n_bits-1), 30)  init_vals=0  sample_rate=1
  simple_bram_vacc : Subsystem  AncestorBlock=casper_library_accumulators/simple_bram_vacc  mask(simple_bram_vacc){vec_len=2^nchan, arith_type=Signed, n_bits=32, bin_pt=30}
      mask prompts: vec_len "Vector length:"; arith_type "Output type:"; n_bits "Bit width (output):"; bin_pt "Binary point (output):"
      mask help: This simple vector accumulator is based on a shift register. It outputs its previous accumulated vector after a new_acc pulse is received.
      mask init:
      | simple_bram_vacc_init(gcb, ...
      |     'vec_len', vec_len, ...
      |     'arith_type', arith_type, ...
      |     'n_bits', n_bits, ...
      |     'bin_pt', bin_pt);
      mask TypeOptions arith_type: Signed | Unsigned
  simple_bram_vacc1 : Subsystem  AncestorBlock=casper_library_accumulators/simple_bram_vacc  mask(simple_bram_vacc){vec_len=2^nchan, arith_type=Signed, n_bits=32, bin_pt=30}
      mask prompts: vec_len "Vector length:"; arith_type "Output type:"; n_bits "Bit width (output):"; bin_pt "Binary point (output):"
      mask help: This simple vector accumulator is based on a shift register. It outputs its previous accumulated vector after a new_acc pulse is received.
      mask init:
      | simple_bram_vacc_init(gcb, ...
      |     'vec_len', vec_len, ...
      |     'arith_type', arith_type, ...
      |     'n_bits', n_bits, ...
      |     'bin_pt', bin_pt);
      mask TypeOptions arith_type: Signed | Unsigned
  wires:
  simple_bram_vacc1/2(valid) -> imag/3
  simple_bram_vacc1/1(dout) -> imag/2
  Delay/1 -> simple_bram_vacc1/1(new_acc), simple_bram_vacc/1(new_acc), Counter/1
  simple_bram_vacc/1(dout) -> real/2
  Counter/1 -> imag/1, real/1
  simple_bram_vacc/2(valid) -> Counter/2, real/3
  new_acc/1 -> Delay/1
  c+di/1 -> c_to_ri2/1
  a+bi/1 -> c_to_ri1/1
  c_to_ri1/1 -> cmult_4bit_em*/1(a)
  c_to_ri1/2 -> cmult_4bit_em*/2(b)
  c_to_ri2/2 -> cmult_4bit_em*/4(d)
  c_to_ri2/1 -> cmult_4bit_em*/3(c)
  cmult_4bit_em*/1(real) -> simple_bram_vacc/2(din)
  cmult_4bit_em*/2(imag) -> simple_bram_vacc1/2(din)

== system spoco6_250/xengine6/df ==
  a+bi : Inport
  c+di : Inport  Port=2
  new_acc : Inport  Port=3
  Counter : xbsIndex_r4/Counter  cnt_type=Free Running  cnt_to=Inf  operation=Up  start_count=0  cnt_by_val=1  arith_type=Unsigned  n_bits=nchan  bin_pt=0  load_pin=off  rst=on  en=on  explicit_period=on  period=1  use_behavioral_HDL=off  implementation=Fabric  dbl_ovrd=off  block_type=counter
  Delay : xbsIndex_r4/Delay  rst=off  infoeditControl=Selection of Reset will increase slice count due to use of real FFs and instead of SRLs  en=off  latency=mult_latency + add_latency  reg_retiming=off  dbl_ovrd=off  block_type=delay
  c_to_ri1 : casper_library_misc/c_to_ri  n_bits=n_bits  bin_pt=n_bits-1
      settings: AttributesFormatString=4_3 r/i
  c_to_ri2 : casper_library_misc/c_to_ri  n_bits=n_bits  bin_pt=n_bits-1
      settings: AttributesFormatString=4_3 r/i
  cmult_4bit_em* : Subsystem  AncestorBlock=casper_library_multipliers/cmult_4bit_em*  mask(cmult_4bit_em*){mult_latency=mult_latency, add_latency=add_latency}
      mask prompts: mult_latency "Mult Latency"; add_latency "Add Latency"
      mask help: Perform a conjugating complex multiplication (a+bi)(c-di)=(ac+bd)+(bc-ad)i. Implements the logic in dedicated multipliers.
      mask Help: eval('xlWeb(''http://casper.berkeley.edu/wiki/Cmult_4bit_em_'')')
  imag : xps_library/Shared BRAM  Tag=xps:bram  arith_type="Signed  (2's comp)"  addr_width=max(nchan,10)  data_width=32  reg_prim_output=off  reg_core_output=off  optimization=Minimum_Area  data_bin_pt=min(2*(n_bits-1), 30)  init_vals=0  sample_rate=1
  real : xps_library/Shared BRAM  Tag=xps:bram  arith_type="Signed  (2's comp)"  addr_width=max(nchan,10)  data_width=32  reg_prim_output=off  reg_core_output=off  optimization=Minimum_Area  data_bin_pt=min(2*(n_bits-1), 30)  init_vals=0  sample_rate=1
  simple_bram_vacc : Subsystem  AncestorBlock=casper_library_accumulators/simple_bram_vacc  mask(simple_bram_vacc){vec_len=2^nchan, arith_type=Signed, n_bits=32, bin_pt=30}
      mask prompts: vec_len "Vector length:"; arith_type "Output type:"; n_bits "Bit width (output):"; bin_pt "Binary point (output):"
      mask help: This simple vector accumulator is based on a shift register. It outputs its previous accumulated vector after a new_acc pulse is received.
      mask init:
      | simple_bram_vacc_init(gcb, ...
      |     'vec_len', vec_len, ...
      |     'arith_type', arith_type, ...
      |     'n_bits', n_bits, ...
      |     'bin_pt', bin_pt);
      mask TypeOptions arith_type: Signed | Unsigned
  simple_bram_vacc1 : Subsystem  AncestorBlock=casper_library_accumulators/simple_bram_vacc  mask(simple_bram_vacc){vec_len=2^nchan, arith_type=Signed, n_bits=32, bin_pt=30}
      mask prompts: vec_len "Vector length:"; arith_type "Output type:"; n_bits "Bit width (output):"; bin_pt "Binary point (output):"
      mask help: This simple vector accumulator is based on a shift register. It outputs its previous accumulated vector after a new_acc pulse is received.
      mask init:
      | simple_bram_vacc_init(gcb, ...
      |     'vec_len', vec_len, ...
      |     'arith_type', arith_type, ...
      |     'n_bits', n_bits, ...
      |     'bin_pt', bin_pt);
      mask TypeOptions arith_type: Signed | Unsigned
  wires:
  cmult_4bit_em*/2(imag) -> simple_bram_vacc1/2(din)
  cmult_4bit_em*/1(real) -> simple_bram_vacc/2(din)
  c_to_ri2/1 -> cmult_4bit_em*/3(c)
  c_to_ri2/2 -> cmult_4bit_em*/4(d)
  c_to_ri1/2 -> cmult_4bit_em*/2(b)
  c_to_ri1/1 -> cmult_4bit_em*/1(a)
  a+bi/1 -> c_to_ri1/1
  c+di/1 -> c_to_ri2/1
  new_acc/1 -> Delay/1
  simple_bram_vacc/2(valid) -> real/3, Counter/2
  Counter/1 -> real/1, imag/1
  simple_bram_vacc/1(dout) -> real/2
  Delay/1 -> Counter/1, simple_bram_vacc/1(new_acc), simple_bram_vacc1/1(new_acc)
  simple_bram_vacc1/1(dout) -> imag/2
  simple_bram_vacc1/2(valid) -> imag/3
